simulink library "MedusaFRHoligramEQ"  (R2022b)
settings: Solver=VariableStepAuto  StartTime=0.0  StopTime=10.0  RelTol=1e-3
undefined symbols (not defined in the file or in its folder): HoligramEQConfig
libraries: FeaturePath x1, PoolIir x1
settings Model: Creator=ud1041536  LastModifiedBy=sc48041
settings SolverCC: AlgebraicLoopSolver=TrustRegion
settings DebuggingCC: UnconnectedInputMsg=warning  UnconnectedOutputMsg=warning  UnconnectedLineMsg=warning  SFMachineParentedDataDiag=warning  ArithmeticOperatorsInVariantConditions=warning
settings ModelReferenceCC: EnableRefExpFcnMdlSchedulingChecks=on
settings SFSimCC: CustomCodeUndefinedFunction=UseInterfaceOnly

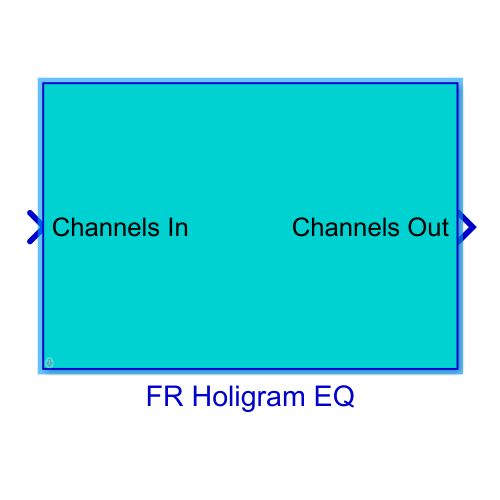
[thumbnail: Simulink's stored preview of the top-level diagram]
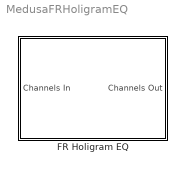
== system MedusaFRHoligramEQ ==
  FR Holigram EQ : Subsystem  mask{configStruct=HoligramEQConfig}
      mask prompts: configStruct "Config struct name:"
      mask init:
      | IIR = configStruct.FRIIR;
      | variantIIR = configStruct.variantIIR;
      | % numOutput = configStruct.numOutput;
      | numOutput = configStruct.numSpkrOutput;
      | frameSize = configStruct.frameSizeFR;
      | 
      | % Construct the IIR Config
      | IirConfig = PoolIirTunableConfig;
      | IirConfig.FrameSize = frameSize;
      | IirConfig.NumChannels = numOutput;
      | IirConfig.MaxNumStages = IIR.maxNumStages;
      | IirConfig.TuneDefaults.NumStages = IIR.numStages;
      | IirConfig.TuneDefaults.SosCoefficients = IIR.coeffs;
      | IirConfig.SelectVariant(variantIIR);
      | IirConfig.Alias = 'HoligramFrIir';
      | 
      | %if(variantIIR == 0)
      | %    IirConfig.SelectVariant('SharcPlusCore');
      | %elseif(variantIIR == 1)
      | %    IirConfig.SelectVariant('SharcPlusAccelGul');
      | %else
      | %    IirConfig.SelectVariant('Generic');
      | %end
      | 
      | % iirBlockPath = MaskUtil.SubBlockName(gcbh, 'IIR');
      | % iirBlockHandle = getSimulinkBlockHandle(iirBlockPath);
      | % if -1 ~= iirBlockHandle
      | %     set_param(iirBlockHandle, 'variantSelect', variantIIR);
      | %     if variantIIR == 1 % Set two extras block params for Accel implementation
      | %         set_param(iirBlockHandle, 'numChannels', num2str(numOutput));
      | %         set_param(iirBlockHandle, 'frameSize', num2str(frameSize));
      | %     end
      | % end

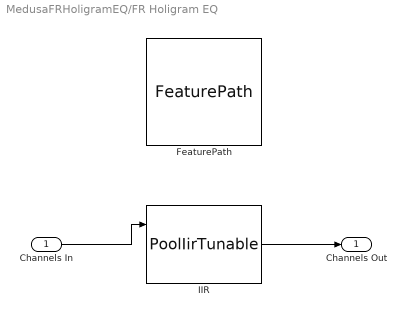
== system MedusaFRHoligramEQ/FR Holigram EQ ==
  Channels In : Inport
  FeaturePath : FeaturePath/FeaturePath  FeatureName=FRHoligram  IsGroup=off  GroupNumber=-1  IsModule=off  TriggerInit=[225 439 340 546]
      settings: SourceProductName=Bose Talaria
  IIR : PoolIir/PoolIirTunable  FeatureName=IirConfig  Config=IirConfig
  Channels Out : Outport  VectorParamsAs1DForOutWhenUnconnected=off
  wires:
  Channels In/1 -> IIR/1
  IIR/1 -> Channels Out/1
